simulink model "Cascade7"  (R2020a)
settings: Solver=FixedStepDiscrete  StartTime=0.0  StopTime=10.0  RelTol=1e-3
settings Model: Creator=DELL  LastModifiedBy=DELL

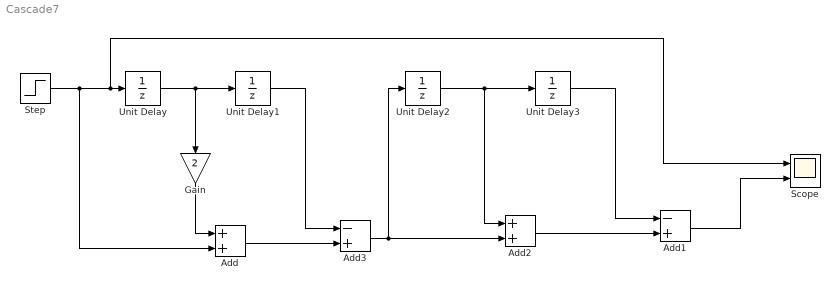
== system Cascade7 ==
  Add : Sum
  Add1 : Sum  Inputs=-+
  Add2 : Sum
  Add3 : Sum  Inputs=-+
  Gain : Gain  Gain=2
  Scope : Scope  NumInputPorts=2
  Step : Step  SampleTime=0
  Unit Delay{,1..3} (4 alike) : UnitDelay  SampleTime=-1  HasFrameUpgradeWarning=on
  wires:
  Step/1 -> Add/2, Scope/1, Unit Delay/1
  Unit Delay/1 -> Gain/1, Unit Delay1/1
  Gain/1 -> Add/1
  Unit Delay1/1 -> Add3/1
  Add/1 -> Add3/2
  Add3/1 -> Add2/2, Unit Delay2/1
  Unit Delay2/1 -> Add2/1, Unit Delay3/1
  Add2/1 -> Add1/2
  Unit Delay3/1 -> Add1/1
  Add1/1 -> Scope/2
